simulink model "rsgTask"  (R2012b)
settings: Solver=FixedStepDiscrete  StartTime=0.0  StopTime=10.0  FixedStep=0.001  RelTol=1e-3
undefined symbols (not defined in the file): acquireMethods, autoplayMovementDuration, autoplayReactionTime, autoplayRotationDuration, autoplayRotationStart, centerOffset, clickPercentage, clickRefractoryPeriod, clickTargetColor, clickTargetHoverColor, clickTargs, coherences, contextIDs, contextTime, contextTimeVec, crossSize, cuedText, cuedTextLength, cumulativeDwell, cursorColorClick, cursorColorClosed, cursorColorOpen, cursorColors, cursorDiameter, cursorNeuralColor, cursorNonneuralColor, delayOrder, delayPeriodGainScale, delayTime, discreteOLMode, displayObject, doHeadSpeedFail, drawNumbersOnTargets, dwellRefractoryPeriod, errorAssistAxis, errorAssistR, errorAssistTheta, expRandBinSize, expRandMax, expRandMin, expRandMu, eyeMode, failOnLiftoff, failurePenalty, falseClickFails, fingerPositionTolerance, fixedSeqMode, freePlayMode, gain, gloveBias, gloveLPDenominator, gloveLPNumerator, gloveNonlinearCorrection, gloveXCorrection, gloveYCorrection, gracePeriod, gridEdges, gridSize, gridTilesEachDim, headSpeedCap ... (+133)
settings Model: Creator=gilja  LastModifiedBy=NPTL
settings SolverCC: EnableConcurrentExecution=on  ConcurrentTasks=on
settings DataIOCC: SaveOutput=off  SignalLogging=off  SaveTime=off
settings OptimizationCC: InlineParams=on  InlineInvariantSignals=on  EnhancedBackFolding=on  EfficientFloat2IntCast=on  SimCompilerOptimization=On
settings DebuggingCC: UnderspecifiedInitializationDetection=Simplified
settings HardwareCC: ProdIntDivRoundTo=Zero  ProdEndianess=LittleEndian  ProdHWDeviceType=Generic->32-bit x86 compatible
settings RTWCC: SystemTargetFile=xpctarget.tlc  TemplateMakefile=xpc_default_tmf  Description=xPC Target  ProcessScript=xpctarget_make_rtw_hook  RTWCompilerOptimization=On
settings CodeAppCC: MaxIdLength=62
settings xpcTargetCC: TargetFcnLib=ansi_tfl_table_tmw.mat  CodeReplacementLibrary=XPC_BLAS  ParMdlRefBuildCompliant=on  ConcurrentExecutionCompliant=on  CombineSignalStateStructs=off  GRTInterface=on  xPCTaskExecutionProfile=on  xPCRL32EventNumber=5000  xPCisDownloadable=off  xPCLoadParamSetFile=off  xPCConcurrentTasks=off  xPCEnableSFAnimation=off

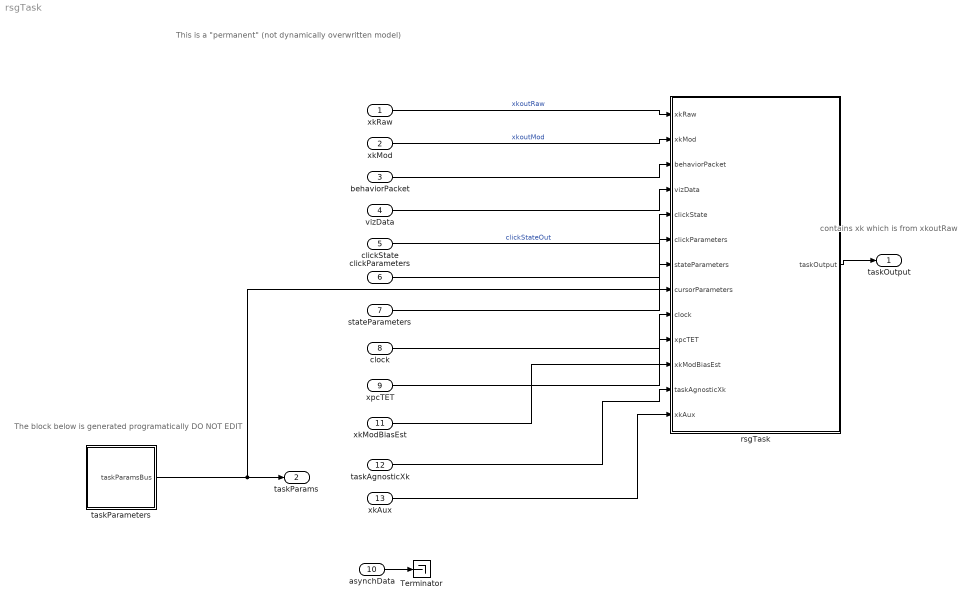
== system rsgTask ==
  note: contains xk which is
      | from xkoutRaw
  note: This is a "permanent" (not dynamically overwritten model)
  note: The block below is generated programatically
      | DO NOT EDIT
  xkRaw : Inport  OutDataTypeStr=double  PortDimensions=[double(xkConstants.NUM_STATE_DIMENSIONS),1]  SampleTime=[0.001,0]
  xkMod : Inport  Port=2  OutDataTypeStr=double  PortDimensions=[double(xkConstants.NUM_STATE_DIMENSIONS),1]  SampleTime=[0.001,0]
  behaviorPacket : Inport  Port=3  OutDataTypeStr=Bus: behaviorPacketBus  SampleTime=[0.001,0]
  vizData : Inport  Port=4  OutDataTypeStr=Bus: peripheralData  SampleTime=[0.001,0]
  clickState : Inport  Port=5  OutDataTypeStr=uint16  PortDimensions=1  SampleTime=[0.001,0]
  clickParameters : Inport  Port=6  OutDataTypeStr=Bus: clickParametersBus  SampleTime=[0.001,0]
  stateParameters : Inport  Port=7  OutDataTypeStr=Bus: stateParams  SampleTime=[0.001,0]
  clock : Inport  Port=8  OutDataTypeStr=uint32  PortDimensions=1  SampleTime=[0.001,0]
  xpcTET : Inport  Port=9  OutDataTypeStr=double  PortDimensions=1  SampleTime=[0.001,0]
  asynchData : Inport  Port=10  OutDataTypeStr=Bus: peripheralData  SampleTime=[0.001,0]
  xkModBiasEst : Inport  Port=11  OutDataTypeStr=double  PortDimensions=[double(xkConstants.NUM_STATE_DIMENSIONS),1]  SampleTime=[0.001,0]
  taskAgnosticXk : Inport  Port=12  OutDataTypeStr=double  PortDimensions=[double(xkConstants.NUM_STATE_DIMENSIONS),1]  SampleTime=[0.001,0]
  xkAux : Inport  Port=13  OutDataTypeStr=double  PortDimensions=[double(xkConstants.NUM_STATE_DIMENSIONS),1]  SampleTime=[0.001,0]
  Terminator : Terminator
  rsgTask : MATLAB Function  TreatAsAtomicUnit=on
  taskParameters : Subsystem
  taskOutput : Outport  OutDataTypeStr=Bus: taskOutput  PortDimensions=1  SampleTime=[0.001,0]  BusOutputAsStruct=on
  taskParams : Outport  Port=2  OutDataTypeStr=Bus: taskParamsBus  SampleTime=[0.001,0]
  wires:
  xkRaw/1 -> rsgTask/1(xkRaw)  "xkoutRaw"
  behaviorPacket/1 -> rsgTask/3(behaviorPacket)
  vizData/1 -> rsgTask/4(vizData)
  clickState/1 -> rsgTask/5(clickState)  "clickStateOut"
  clickParameters/1 -> rsgTask/6(clickParameters)
  clock/1 -> rsgTask/9(clock)
  xpcTET/1 -> rsgTask/10(xpcTET)
  stateParameters/1 -> rsgTask/7(stateParameters)
  taskParameters/1(taskParamsBus) -> taskParams/1, rsgTask/8(cursorParameters)
  rsgTask/1(taskOutput) -> taskOutput/1
  asynchData/1 -> Terminator/1
  xkMod/1 -> rsgTask/2(xkMod)  "xkoutMod"
  xkModBiasEst/1 -> rsgTask/11(xkModBiasEst)
  taskAgnosticXk/1 -> rsgTask/12(taskAgnosticXk)
  xkAux/1 -> rsgTask/13(xkAux)

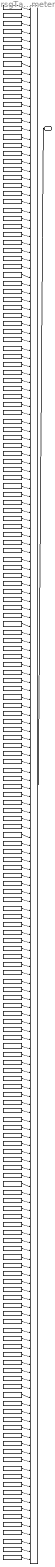
== system rsgTask/taskParameters ==
  BusOutput : BusCreator  Inputs=targetDiameter,maxTaskTime,holdTime,trialTimeout,numTrials,randomSeed,expRandMu,expRandMin,expRandMax,expRandBinSize,taskType,targetInds,numTargets,gain,failurePenalty,cursorDiameter,inputType,gloveBias,useRandomDelay,mouseOffset,workspaceX,workspaceY,workspaceZ,workspaceR,workspaceR2,showScores,trialsPerScore,cursorColorClick,recenterOnFail,recenterOnSuccess,recenterDelay,initialInput,clickPercentage,lockFingerPosition,fingerPositionTolerance,failOnLiftoff,errorAssistR,errorAssistTheta,errorAssistAxis,useGloveLPF,gloveLPNumerator,gloveLPDenominator,gloveNonlinearCorrection,gloveYCorrection,gloveXCorrection,useMouseLPF,soundOnFail,soundOnGo,soundOnSuccess,soundOnOverTarget,mouseLPNumerator,mouseLPDenominator,stopOffTarget,stopOnClick,outputType,xk2HorizontalPos,xk2HorizontalVel,xk2VerticalPos,xk2VerticalVel,xk2DepthPos,xk2DepthVel,xk2RotatePos,xk2RotateVel,xk2Rotate2Pos,xk2Rotate2Vel,gridEdges,gridTilesEachDim,selectionRefractoryMS,autoplayReactionTime,autoplayMovementDuration,powerGain,powerGainUnityCrossing,targetRotDiameter,autoplayRotationStart,autoplayRotationDuration,randomTaskTargetDiameters,randomTaskTargetRotDiameters,randomTaskBoundaries,numDisplayDims,cursorColorOpen,cursorColorClosed,showXYZaura,displayObject,preTrialLength,targetDiameters,numTargetDiameters,minTargetDistance,targetDelay,targetSpaceX,targetSpaceY,clickTargetColor,clickTargetHoverColor,falseClickFails,splitDimensions,vmrTheta,doHeadSpeedFail,headSpeedCap,eyeMode,speedTaskMode,delayPeriodGainScale,wiaMode,showWiaText,freePlayMode,drawNumbersOnTargets,xkRawSpeedCap,discreteOLMode,movementDuration,holdDuration,restDuration,returnDuration,repsPerBlock,whichMovements,movementOrder,delayOrder,textOverlayID,clickRefractoryPeriod,xpcVelocityOutputPeriodMS,outputVelocityScaling,screenUpdateRate,targetDevice,playSpokenCues,numTargetsInSeq,targetSeq,seqReadyTime,seqRehearseTime,rotateSeqCues,numRepsPerSeq,rehearsalOrder,rehearsalTimes,pathMode,memorizeMode,fixedSeqMode,sequenceMatrix,keyboard,resetDisplay,cursorNeuralColor,cursorNonneuralColor,centerOffset,scoreTime,cuedTextLength,cuedText,keyboardDims,recenterFullscreen,soundOnError,acquireMethods,cumulativeDwell,showBackspace,showStartStop,showTargetText,showTypedText,showCueOnTarget,showCueOffTarget,recenterOffset,dwellRefractoryPeriod,keyPressedTime,initialLockout,initialState,symbolMoveTimeOne,symbolRehearseTime,symbolGetReadyTime,symbolMoveTimeTwo,symbolVMRMode,symbolVMRRot,pc1MouseInControlMode,gracePeriod,maxFixDur,maxTargDur,maxStimDur,moveThresh,intertrialTime,cursorColors,gridSize,crossSize,makeGrid,tau,taskOrder,stimDur,coherences,contextIDs,stimConds,contextTime,stimTime,delayTime,contextTimeVec,nextClickTarg,clickTargs,rsgTargetSeq,rsgTargetLoc,rsgCueDisplayTime,rsgProductionTimes,rsgPreReadyTimes,rsgFixationRadius  OutDataTypeStr=Bus: taskParamsBus
  acquireMethods : Constant  Value=acquireMethods
  autoplayMovementDuration : Constant  Value=autoplayMovementDuration
  autoplayReactionTime : Constant  Value=autoplayReactionTime
  autoplayRotationDuration : Constant  Value=autoplayRotationDuration
  autoplayRotationStart : Constant  Value=autoplayRotationStart
  centerOffset : Constant  Value=centerOffset
  clickPercentage : Constant  Value=clickPercentage
  clickRefractoryPeriod : Constant  Value=clickRefractoryPeriod
  clickTargetColor : Constant  Value=clickTargetColor
  clickTargetHoverColor : Constant  Value=clickTargetHoverColor
  clickTargs : Constant  Value=clickTargs
  coherences : Constant  Value=coherences
  contextIDs : Constant  Value=contextIDs
  contextTime : Constant  Value=contextTime
  contextTimeVec : Constant  Value=contextTimeVec
  crossSize : Constant  Value=crossSize
  cuedText : Constant  Value=cuedText
  cuedTextLength : Constant  Value=cuedTextLength
  cumulativeDwell : Constant  Value=cumulativeDwell
  cursorColorClick : Constant  Value=cursorColorClick
  cursorColorClosed : Constant  Value=cursorColorClosed
  cursorColorOpen : Constant  Value=cursorColorOpen
  cursorColors : Constant  Value=cursorColors
  cursorDiameter : Constant  Value=cursorDiameter
  cursorNeuralColor : Constant  Value=cursorNeuralColor
  cursorNonneuralColor : Constant  Value=cursorNonneuralColor
  delayOrder : Constant  Value=delayOrder
  delayPeriodGainScale : Constant  Value=delayPeriodGainScale
  delayTime : Constant  Value=delayTime
  discreteOLMode : Constant  Value=discreteOLMode
  displayObject : Constant  Value=displayObject
  doHeadSpeedFail : Constant  Value=doHeadSpeedFail
  drawNumbersOnTargets : Constant  Value=drawNumbersOnTargets
  dwellRefractoryPeriod : Constant  Value=dwellRefractoryPeriod
  errorAssistAxis : Constant  Value=errorAssistAxis
  errorAssistR : Constant  Value=errorAssistR
  errorAssistTheta : Constant  Value=errorAssistTheta
  expRandBinSize : Constant  Value=expRandBinSize
  expRandMax : Constant  Value=expRandMax
  expRandMin : Constant  Value=expRandMin
  expRandMu : Constant  Value=expRandMu
  eyeMode : Constant  Value=eyeMode
  failOnLiftoff : Constant  Value=failOnLiftoff
  failurePenalty : Constant  Value=failurePenalty
  falseClickFails : Constant  Value=falseClickFails
  fingerPositionTolerance : Constant  Value=fingerPositionTolerance
  fixedSeqMode : Constant  Value=fixedSeqMode
  freePlayMode : Constant  Value=freePlayMode
  gain : Constant  Value=gain
  gloveBias : Constant  Value=gloveBias
  gloveLPDenominator : Constant  Value=gloveLPDenominator
  gloveLPNumerator : Constant  Value=gloveLPNumerator
  gloveNonlinearCorrection : Constant  Value=gloveNonlinearCorrection
  gloveXCorrection : Constant  Value=gloveXCorrection
  gloveYCorrection : Constant  Value=gloveYCorrection
  gracePeriod : Constant  Value=gracePeriod
  gridEdges : Constant  Value=gridEdges
  gridSize : Constant  Value=gridSize
  gridTilesEachDim : Constant  Value=gridTilesEachDim
  headSpeedCap : Constant  Value=headSpeedCap
  holdDuration : Constant  Value=holdDuration
  holdTime : Constant  Value=holdTime
  initialInput : Constant  Value=initialInput
  initialLockout : Constant  Value=initialLockout
  initialState : Constant  Value=initialState
  inputType : Constant  Value=inputType
  intertrialTime : Constant  Value=intertrialTime
  keyPressedTime : Constant  Value=keyPressedTime
  keyboard : Constant  Value=keyboard
  keyboardDims : Constant  Value=keyboardDims
  lockFingerPosition : Constant  Value=lockFingerPosition
  makeGrid : Constant  Value=makeGrid
  maxFixDur : Constant  Value=maxFixDur
  maxStimDur : Constant  Value=maxStimDur
  maxTargDur : Constant  Value=maxTargDur
  maxTaskTime : Constant  Value=maxTaskTime
  memorizeMode : Constant  Value=memorizeMode
  minTargetDistance : Constant  Value=minTargetDistance
  mouseLPDenominator : Constant  Value=mouseLPDenominator
  mouseLPNumerator : Constant  Value=mouseLPNumerator
  mouseOffset : Constant  Value=mouseOffset
  moveThresh : Constant  Value=moveThresh
  movementDuration : Constant  Value=movementDuration
  movementOrder : Constant  Value=movementOrder
  nextClickTarg : Constant  Value=nextClickTarg
  numDisplayDims : Constant  Value=numDisplayDims
  numRepsPerSeq : Constant  Value=numRepsPerSeq
  numTargetDiameters : Constant  Value=numTargetDiameters
  numTargets : Constant  Value=numTargets
  numTargetsInSeq : Constant  Value=numTargetsInSeq
  numTrials : Constant  Value=numTrials
  outputType : Constant  Value=outputType
  outputVelocityScaling : Constant  Value=outputVelocityScaling
  pathMode : Constant  Value=pathMode
  pc1MouseInControlMode : Constant  Value=pc1MouseInControlMode
  playSpokenCues : Constant  Value=playSpokenCues
  powerGain : Constant  Value=powerGain
  powerGainUnityCrossing : Constant  Value=powerGainUnityCrossing
  preTrialLength : Constant  Value=preTrialLength
  randomSeed : Constant  Value=randomSeed
  randomTaskBoundaries : Constant  Value=randomTaskBoundaries
  randomTaskTargetDiameters : Constant  Value=randomTaskTargetDiameters
  randomTaskTargetRotDiameters : Constant  Value=randomTaskTargetRotDiameters
  recenterDelay : Constant  Value=recenterDelay
  recenterFullscreen : Constant  Value=recenterFullscreen
  recenterOffset : Constant  Value=recenterOffset
  recenterOnFail : Constant  Value=recenterOnFail
  recenterOnSuccess : Constant  Value=recenterOnSuccess
  rehearsalOrder : Constant  Value=rehearsalOrder
  rehearsalTimes : Constant  Value=rehearsalTimes
  repsPerBlock : Constant  Value=repsPerBlock
  resetDisplay : Constant  Value=resetDisplay
  restDuration : Constant  Value=restDuration
  returnDuration : Constant  Value=returnDuration
  rotateSeqCues : Constant  Value=rotateSeqCues
  rsgCueDisplayTime : Constant  Value=rsgCueDisplayTime
  rsgFixationRadius : Constant  Value=rsgFixationRadius
  rsgPreReadyTimes : Constant  Value=rsgPreReadyTimes
  rsgProductionTimes : Constant  Value=rsgProductionTimes
  rsgTargetLoc : Constant  Value=rsgTargetLoc
  rsgTargetSeq : Constant  Value=rsgTargetSeq
  scoreTime : Constant  Value=scoreTime
  screenUpdateRate : Constant  Value=screenUpdateRate
  selectionRefractoryMS : Constant  Value=selectionRefractoryMS
  seqReadyTime : Constant  Value=seqReadyTime
  seqRehearseTime : Constant  Value=seqRehearseTime
  sequenceMatrix : Constant  Value=sequenceMatrix
  showBackspace : Constant  Value=showBackspace
  showCueOffTarget : Constant  Value=showCueOffTarget
  showCueOnTarget : Constant  Value=showCueOnTarget
  showScores : Constant  Value=showScores
  showStartStop : Constant  Value=showStartStop
  showTargetText : Constant  Value=showTargetText
  showTypedText : Constant  Value=showTypedText
  showWiaText : Constant  Value=showWiaText
  showXYZaura : Constant  Value=showXYZaura
  soundOnError : Constant  Value=soundOnError
  soundOnFail : Constant  Value=soundOnFail
  soundOnGo : Constant  Value=soundOnGo
  soundOnOverTarget : Constant  Value=soundOnOverTarget
  soundOnSuccess : Constant  Value=soundOnSuccess
  speedTaskMode : Constant  Value=speedTaskMode
  splitDimensions : Constant  Value=splitDimensions
  stimConds : Constant  Value=stimConds
  stimDur : Constant  Value=stimDur
  stimTime : Constant  Value=stimTime
  stopOffTarget : Constant  Value=stopOffTarget
  stopOnClick : Constant  Value=stopOnClick
  symbolGetReadyTime : Constant  Value=symbolGetReadyTime
  symbolMoveTimeOne : Constant  Value=symbolMoveTimeOne
  symbolMoveTimeTwo : Constant  Value=symbolMoveTimeTwo
  symbolRehearseTime : Constant  Value=symbolRehearseTime
  symbolVMRMode : Constant  Value=symbolVMRMode
  symbolVMRRot : Constant  Value=symbolVMRRot
  targetDelay : Constant  Value=targetDelay
  targetDevice : Constant  Value=targetDevice
  targetDiameter : Constant  Value=targetDiameter
  targetDiameters : Constant  Value=targetDiameters
  targetInds : Constant  Value=targetInds
  targetRotDiameter : Constant  Value=targetRotDiameter
  targetSeq : Constant  Value=targetSeq
  targetSpaceX : Constant  Value=targetSpaceX
  targetSpaceY : Constant  Value=targetSpaceY
  taskOrder : Constant  Value=taskOrder
  taskType : Constant  Value=taskType
  tau : Constant  Value=tau
  textOverlayID : Constant  Value=textOverlayID
  trialTimeout : Constant  Value=trialTimeout
  trialsPerScore : Constant  Value=trialsPerScore
  useGloveLPF : Constant  Value=useGloveLPF
  useMouseLPF : Constant  Value=useMouseLPF
  useRandomDelay : Constant  Value=useRandomDelay
  vmrTheta : Constant  Value=vmrTheta
  whichMovements : Constant  Value=whichMovements
  wiaMode : Constant  Value=wiaMode
  workspaceR : Constant  Value=workspaceR
  workspaceR2 : Constant  Value=workspaceR2
  workspaceX : Constant  Value=workspaceX
  workspaceY : Constant  Value=workspaceY
  workspaceZ : Constant  Value=workspaceZ
  xk2DepthPos : Constant  Value=xk2DepthPos
  xk2DepthVel : Constant  Value=xk2DepthVel
  xk2HorizontalPos : Constant  Value=xk2HorizontalPos
  xk2HorizontalVel : Constant  Value=xk2HorizontalVel
  xk2Rotate2Pos : Constant  Value=xk2Rotate2Pos
  xk2Rotate2Vel : Constant  Value=xk2Rotate2Vel
  xk2RotatePos : Constant  Value=xk2RotatePos
  xk2RotateVel : Constant  Value=xk2RotateVel
  xk2VerticalPos : Constant  Value=xk2VerticalPos
  xk2VerticalVel : Constant  Value=xk2VerticalVel
  xkRawSpeedCap : Constant  Value=xkRawSpeedCap
  xpcVelocityOutputPeriodMS : Constant  Value=xpcVelocityOutputPeriodMS
  taskParamsBus : Outport
  wires:
  targetDiameter/1 -> BusOutput/1  "targetDiameter"
  maxTaskTime/1 -> BusOutput/2  "maxTaskTime"
  holdTime/1 -> BusOutput/3  "holdTime"
  trialTimeout/1 -> BusOutput/4  "trialTimeout"
  numTrials/1 -> BusOutput/5  "numTrials"
  randomSeed/1 -> BusOutput/6  "randomSeed"
  expRandMu/1 -> BusOutput/7  "expRandMu"
  expRandMin/1 -> BusOutput/8  "expRandMin"
  expRandMax/1 -> BusOutput/9  "expRandMax"
  expRandBinSize/1 -> BusOutput/10  "expRandBinSize"
  taskType/1 -> BusOutput/11  "taskType"
  targetInds/1 -> BusOutput/12  "targetInds"
  numTargets/1 -> BusOutput/13  "numTargets"
  gain/1 -> BusOutput/14  "gain"
  failurePenalty/1 -> BusOutput/15  "failurePenalty"
  cursorDiameter/1 -> BusOutput/16  "cursorDiameter"
  inputType/1 -> BusOutput/17  "inputType"
  gloveBias/1 -> BusOutput/18  "gloveBias"
  useRandomDelay/1 -> BusOutput/19  "useRandomDelay"
  mouseOffset/1 -> BusOutput/20  "mouseOffset"
  workspaceX/1 -> BusOutput/21  "workspaceX"
  workspaceY/1 -> BusOutput/22  "workspaceY"
  workspaceZ/1 -> BusOutput/23  "workspaceZ"
  workspaceR/1 -> BusOutput/24  "workspaceR"
  workspaceR2/1 -> BusOutput/25  "workspaceR2"
  showScores/1 -> BusOutput/26  "showScores"
  trialsPerScore/1 -> BusOutput/27  "trialsPerScore"
  cursorColorClick/1 -> BusOutput/28  "cursorColorClick"
  recenterOnFail/1 -> BusOutput/29  "recenterOnFail"
  recenterOnSuccess/1 -> BusOutput/30  "recenterOnSuccess"
  recenterDelay/1 -> BusOutput/31  "recenterDelay"
  initialInput/1 -> BusOutput/32  "initialInput"
  clickPercentage/1 -> BusOutput/33  "clickPercentage"
  lockFingerPosition/1 -> BusOutput/34  "lockFingerPosition"
  fingerPositionTolerance/1 -> BusOutput/35  "fingerPositionTolerance"
  failOnLiftoff/1 -> BusOutput/36  "failOnLiftoff"
  errorAssistR/1 -> BusOutput/37  "errorAssistR"
  errorAssistTheta/1 -> BusOutput/38  "errorAssistTheta"
  errorAssistAxis/1 -> BusOutput/39  "errorAssistAxis"
  useGloveLPF/1 -> BusOutput/40  "useGloveLPF"
  gloveLPNumerator/1 -> BusOutput/41  "gloveLPNumerator"
  gloveLPDenominator/1 -> BusOutput/42  "gloveLPDenominator"
  gloveNonlinearCorrection/1 -> BusOutput/43  "gloveNonlinearCorrection"
  gloveYCorrection/1 -> BusOutput/44  "gloveYCorrection"
  gloveXCorrection/1 -> BusOutput/45  "gloveXCorrection"
  useMouseLPF/1 -> BusOutput/46  "useMouseLPF"
  soundOnFail/1 -> BusOutput/47  "soundOnFail"
  soundOnGo/1 -> BusOutput/48  "soundOnGo"
  soundOnSuccess/1 -> BusOutput/49  "soundOnSuccess"
  soundOnOverTarget/1 -> BusOutput/50  "soundOnOverTarget"
  mouseLPNumerator/1 -> BusOutput/51  "mouseLPNumerator"
  mouseLPDenominator/1 -> BusOutput/52  "mouseLPDenominator"
  stopOffTarget/1 -> BusOutput/53  "stopOffTarget"
  stopOnClick/1 -> BusOutput/54  "stopOnClick"
  outputType/1 -> BusOutput/55  "outputType"
  xk2HorizontalPos/1 -> BusOutput/56  "xk2HorizontalPos"
  xk2HorizontalVel/1 -> BusOutput/57  "xk2HorizontalVel"
  xk2VerticalPos/1 -> BusOutput/58  "xk2VerticalPos"
  xk2VerticalVel/1 -> BusOutput/59  "xk2VerticalVel"
  xk2DepthPos/1 -> BusOutput/60  "xk2DepthPos"
  xk2DepthVel/1 -> BusOutput/61  "xk2DepthVel"
  xk2RotatePos/1 -> BusOutput/62  "xk2RotatePos"
  xk2RotateVel/1 -> BusOutput/63  "xk2RotateVel"
  xk2Rotate2Pos/1 -> BusOutput/64  "xk2Rotate2Pos"
  xk2Rotate2Vel/1 -> BusOutput/65  "xk2Rotate2Vel"
  gridEdges/1 -> BusOutput/66  "gridEdges"
  gridTilesEachDim/1 -> BusOutput/67  "gridTilesEachDim"
  selectionRefractoryMS/1 -> BusOutput/68  "selectionRefractoryMS"
  autoplayReactionTime/1 -> BusOutput/69  "autoplayReactionTime"
  autoplayMovementDuration/1 -> BusOutput/70  "autoplayMovementDuration"
  powerGain/1 -> BusOutput/71  "powerGain"
  powerGainUnityCrossing/1 -> BusOutput/72  "powerGainUnityCrossing"
  targetRotDiameter/1 -> BusOutput/73  "targetRotDiameter"
  autoplayRotationStart/1 -> BusOutput/74  "autoplayRotationStart"
  autoplayRotationDuration/1 -> BusOutput/75  "autoplayRotationDuration"
  randomTaskTargetDiameters/1 -> BusOutput/76  "randomTaskTargetDiameters"
  randomTaskTargetRotDiameters/1 -> BusOutput/77  "randomTaskTargetRotDiameters"
  randomTaskBoundaries/1 -> BusOutput/78  "randomTaskBoundaries"
  numDisplayDims/1 -> BusOutput/79  "numDisplayDims"
  cursorColorOpen/1 -> BusOutput/80  "cursorColorOpen"
  cursorColorClosed/1 -> BusOutput/81  "cursorColorClosed"
  showXYZaura/1 -> BusOutput/82  "showXYZaura"
  displayObject/1 -> BusOutput/83  "displayObject"
  preTrialLength/1 -> BusOutput/84  "preTrialLength"
  targetDiameters/1 -> BusOutput/85  "targetDiameters"
  numTargetDiameters/1 -> BusOutput/86  "numTargetDiameters"
  minTargetDistance/1 -> BusOutput/87  "minTargetDistance"
  targetDelay/1 -> BusOutput/88  "targetDelay"
  targetSpaceX/1 -> BusOutput/89  "targetSpaceX"
  targetSpaceY/1 -> BusOutput/90  "targetSpaceY"
  clickTargetColor/1 -> BusOutput/91  "clickTargetColor"
  clickTargetHoverColor/1 -> BusOutput/92  "clickTargetHoverColor"
  falseClickFails/1 -> BusOutput/93  "falseClickFails"
  splitDimensions/1 -> BusOutput/94  "splitDimensions"
  vmrTheta/1 -> BusOutput/95  "vmrTheta"
  doHeadSpeedFail/1 -> BusOutput/96  "doHeadSpeedFail"
  headSpeedCap/1 -> BusOutput/97  "headSpeedCap"
  eyeMode/1 -> BusOutput/98  "eyeMode"
  speedTaskMode/1 -> BusOutput/99  "speedTaskMode"
  delayPeriodGainScale/1 -> BusOutput/100  "delayPeriodGainScale"
  wiaMode/1 -> BusOutput/101  "wiaMode"
  showWiaText/1 -> BusOutput/102  "showWiaText"
  freePlayMode/1 -> BusOutput/103  "freePlayMode"
  drawNumbersOnTargets/1 -> BusOutput/104  "drawNumbersOnTargets"
  xkRawSpeedCap/1 -> BusOutput/105  "xkRawSpeedCap"
  discreteOLMode/1 -> BusOutput/106  "discreteOLMode"
  movementDuration/1 -> BusOutput/107  "movementDuration"
  holdDuration/1 -> BusOutput/108  "holdDuration"
  restDuration/1 -> BusOutput/109  "restDuration"
  returnDuration/1 -> BusOutput/110  "returnDuration"
  repsPerBlock/1 -> BusOutput/111  "repsPerBlock"
  whichMovements/1 -> BusOutput/112  "whichMovements"
  movementOrder/1 -> BusOutput/113  "movementOrder"
  delayOrder/1 -> BusOutput/114  "delayOrder"
  textOverlayID/1 -> BusOutput/115  "textOverlayID"
  clickRefractoryPeriod/1 -> BusOutput/116  "clickRefractoryPeriod"
  xpcVelocityOutputPeriodMS/1 -> BusOutput/117  "xpcVelocityOutputPeriodMS"
  outputVelocityScaling/1 -> BusOutput/118  "outputVelocityScaling"
  screenUpdateRate/1 -> BusOutput/119  "screenUpdateRate"
  targetDevice/1 -> BusOutput/120  "targetDevice"
  playSpokenCues/1 -> BusOutput/121  "playSpokenCues"
  numTargetsInSeq/1 -> BusOutput/122  "numTargetsInSeq"
  targetSeq/1 -> BusOutput/123  "targetSeq"
  seqReadyTime/1 -> BusOutput/124  "seqReadyTime"
  seqRehearseTime/1 -> BusOutput/125  "seqRehearseTime"
  rotateSeqCues/1 -> BusOutput/126  "rotateSeqCues"
  numRepsPerSeq/1 -> BusOutput/127  "numRepsPerSeq"
  rehearsalOrder/1 -> BusOutput/128  "rehearsalOrder"
  rehearsalTimes/1 -> BusOutput/129  "rehearsalTimes"
  pathMode/1 -> BusOutput/130  "pathMode"
  memorizeMode/1 -> BusOutput/131  "memorizeMode"
  fixedSeqMode/1 -> BusOutput/132  "fixedSeqMode"
  sequenceMatrix/1 -> BusOutput/133  "sequenceMatrix"
  keyboard/1 -> BusOutput/134  "keyboard"
  resetDisplay/1 -> BusOutput/135  "resetDisplay"
  cursorNeuralColor/1 -> BusOutput/136  "cursorNeuralColor"
  cursorNonneuralColor/1 -> BusOutput/137  "cursorNonneuralColor"
  centerOffset/1 -> BusOutput/138  "centerOffset"
  scoreTime/1 -> BusOutput/139  "scoreTime"
  cuedTextLength/1 -> BusOutput/140  "cuedTextLength"
  cuedText/1 -> BusOutput/141  "cuedText"
  keyboardDims/1 -> BusOutput/142  "keyboardDims"
  recenterFullscreen/1 -> BusOutput/143  "recenterFullscreen"
  soundOnError/1 -> BusOutput/144  "soundOnError"
  acquireMethods/1 -> BusOutput/145  "acquireMethods"
  cumulativeDwell/1 -> BusOutput/146  "cumulativeDwell"
  showBackspace/1 -> BusOutput/147  "showBackspace"
  showStartStop/1 -> BusOutput/148  "showStartStop"
  showTargetText/1 -> BusOutput/149  "showTargetText"
  showTypedText/1 -> BusOutput/150  "showTypedText"
  showCueOnTarget/1 -> BusOutput/151  "showCueOnTarget"
  showCueOffTarget/1 -> BusOutput/152  "showCueOffTarget"
  recenterOffset/1 -> BusOutput/153  "recenterOffset"
  dwellRefractoryPeriod/1 -> BusOutput/154  "dwellRefractoryPeriod"
  keyPressedTime/1 -> BusOutput/155  "keyPressedTime"
  initialLockout/1 -> BusOutput/156  "initialLockout"
  initialState/1 -> BusOutput/157  "initialState"
  symbolMoveTimeOne/1 -> BusOutput/158  "symbolMoveTimeOne"
  symbolRehearseTime/1 -> BusOutput/159  "symbolRehearseTime"
  symbolGetReadyTime/1 -> BusOutput/160  "symbolGetReadyTime"
  symbolMoveTimeTwo/1 -> BusOutput/161  "symbolMoveTimeTwo"
  symbolVMRMode/1 -> BusOutput/162  "symbolVMRMode"
  symbolVMRRot/1 -> BusOutput/163  "symbolVMRRot"
  pc1MouseInControlMode/1 -> BusOutput/164  "pc1MouseInControlMode"
  gracePeriod/1 -> BusOutput/165  "gracePeriod"
  maxFixDur/1 -> BusOutput/166  "maxFixDur"
  maxTargDur/1 -> BusOutput/167  "maxTargDur"
  maxStimDur/1 -> BusOutput/168  "maxStimDur"
  moveThresh/1 -> BusOutput/169  "moveThresh"
  intertrialTime/1 -> BusOutput/170  "intertrialTime"
  cursorColors/1 -> BusOutput/171  "cursorColors"
  gridSize/1 -> BusOutput/172  "gridSize"
  crossSize/1 -> BusOutput/173  "crossSize"
  makeGrid/1 -> BusOutput/174  "makeGrid"
  tau/1 -> BusOutput/175  "tau"
  taskOrder/1 -> BusOutput/176  "taskOrder"
  stimDur/1 -> BusOutput/177  "stimDur"
  coherences/1 -> BusOutput/178  "coherences"
  contextIDs/1 -> BusOutput/179  "contextIDs"
  stimConds/1 -> BusOutput/180  "stimConds"
  contextTime/1 -> BusOutput/181  "contextTime"
  stimTime/1 -> BusOutput/182  "stimTime"
  delayTime/1 -> BusOutput/183  "delayTime"
  contextTimeVec/1 -> BusOutput/184  "contextTimeVec"
  nextClickTarg/1 -> BusOutput/185  "nextClickTarg"
  clickTargs/1 -> BusOutput/186  "clickTargs"
  rsgTargetSeq/1 -> BusOutput/187  "rsgTargetSeq"
  rsgTargetLoc/1 -> BusOutput/188  "rsgTargetLoc"
  rsgCueDisplayTime/1 -> BusOutput/189  "rsgCueDisplayTime"
  rsgProductionTimes/1 -> BusOutput/190  "rsgProductionTimes"
  rsgPreReadyTimes/1 -> BusOutput/191  "rsgPreReadyTimes"
  rsgFixationRadius/1 -> BusOutput/192  "rsgFixationRadius"
  BusOutput/1 -> taskParamsBus/1

== matlab function rsgTask/rsgTask ==
  data: xkRaw input double size=[double(xkConstants.NUM_STATE_DIMENSIONS) 1]; xkMod input; behaviorPacket input Bus: behaviorPacketBus size=1; vizData input Bus: peripheralData; clickState input; clickParameters input; taskOutput output Bus: taskOutput; stateParameters input Bus: stateParams size=1; cursorParameters input Bus: taskParamsBus; clock input; xpcTET input; xkModBiasEst input; taskAgnosticXk input; xkAux input
function taskOutput  = rsgTask(xkRaw, xkMod, behaviorPacket, vizData, clickState, clickParameters, ...
    stateParameters, cursorParameters, clock, xpcTET, xkModBiasEst, taskAgnosticXk, xkAux)

%#codegen
behaviorRequestClock = behaviorPacket.xpcRequestClock;
peripheralTimestamp = behaviorPacket.peripheralTimestamp(1:16);

%% CONSTANTS
TASK_NAME = 'rsg';
VERSION_ID = single(1.0);

%% INITIALIZE CURSOR TASK OUTPUT
fileLoggerData.data = uint8(zeros(1,1400));
fileLoggerData.dataLen = uint16(0);
fileLoggerData.fileName = uint8(zeros(1,20));
fileLoggerData.send = false;

fileLoggerFormat.format = uint8(zeros(1,1400));
fileLoggerFormat.formatLen = uint16(0);
fileLoggerFormat.fileName = uint8(zeros(1,20));

fileLoggerFormatAndData.format = fileLoggerFormat;
fileLoggerFormatAndData.data = fileLoggerData;

taskOutput.flushFiles = false;
taskOutput.sendFormat = false;
taskOutput.taskDetails = fileLoggerFormat;
taskOutput.discrete = fileLoggerFormatAndData;
taskOutput.continuous = fileLoggerFormatAndData;
taskOutput.screen = fileLoggerFormatAndData;
taskOutput.sound = fileLoggerFormatAndData;
taskOutput.asynch = fileLoggerFormatAndData;
taskOutput.ttl = double(0);
taskOutput.xk = xkRaw;
taskOutput.inputType = cursorParameters.inputType;
taskOutput.currentTarget = single(zeros([double(xkConstants.NUM_TARGET_DIMENSIONS) 1]));
taskOutput.state = uint16(SequenceStates.STATE_MOVE);
taskOutput.paused = false;
taskOutput.allowStop = true;
taskOutput.resetHMM = true;

%% TASK DETAILS PACKET
taskOutput.taskDetails = packFileLoggerTaskDetails(TASK_NAME, VERSION_ID, ...
    'STATE_INIT', uint8(rsgStates.STATE_INIT), ...
    'STATE_FIXATE', uint8(rsgStates.STATE_FIXATE),...
    'STATE_PRE_READY', uint8(rsgStates.STATE_PRE_READY),...
    'STATE_POST_READY', uint8(rsgStates.STATE_POST_READY), ...
    'STATE_POST_SET', uint8(rsgStates.STATE_POST_SET),...
    'STATE_ACQUIRE', uint8(rsgStates.STATE_ACQUIRE),...
    'INPUT_TYPE_DECODE_V', uint8(cursorConstants.INPUT_TYPE_DECODE_V),...
    'INPUT_TYPE_HEAD_MOUSE', uint8(cursorConstants.INPUT_TYPE_HEAD_MOUSE) ...
);

%% DEFINE PERSISTENTS
persistent holdTimer 
persistent stateTimer;
persistent trialIdx;
persistent avgErr;
persistent totalErr;
persistent percentErr;
persistent state;

persistent lastSoundTime;
persistent lastSoundState;
persistent vizPacket;
persistent pastPause;

persistent prevHeadPos;
persistent filteredHeadSpeed;

persistent err;
persistent producedTime;
persistent currentTargIdx;

%% INITIALIZE PERSISTENTS
if(isempty(holdTimer))
    holdTimer = uint16(0);
    stateTimer = uint32(0);
    trialIdx = uint32(1);
    avgErr = single(0);
    totalErr = single(0);
    currentTargIdx = uint32(1);

    state = uint8(rsgStates.STATE_INIT);
    prevHeadPos = single(zeros(2,1));
    filteredHeadSpeed = single(0);

    lastSoundTime = clock;
    lastSoundState = uint8(SequenceStates.SOUND_STATE_IDLE);

    vizPacket = initVizPacket();
    pastPause = false;
    
    err = int32(-5000);
    producedTime = int32(-5000);
end
inputType = cursorParameters.inputType;

%% some initialization
outputType = cursorParameters.outputType; % determines what graphics engine will render this task.

writeDiscreteData = false;
writeContinuousData = true;

if(vizData.receive && (vizData.dataLen > 0 ))
    vizPacket = parseVizPacket(vizData.data);
end

effectorPos = zeros(1,2);
effectorPos(1) = behaviorPacket.windowsMousePosition(1)*1080;
effectorPos(2) = -behaviorPacket.windowsMousePosition(2)*1080;

INIT_TIME = uint32(2000);
pauseToggled = (pastPause==true) && (stateParameters.pause==false);
pauseTriggered = stateParameters.pause;
pastPause = stateParameters.pause;

if(clock < INIT_TIME)
    state = uint8(rsgStates.STATE_INIT);
    pauseTriggered = true;
elseif (state == uint8(rsgStates.STATE_INIT)) && pauseToggled
    state = uint8(rsgStates.STATE_FIXATE);
    stateTimer = uint32(1);
    trialIdx = uint32(0);
end

%%
%continuously affect state of RNG so we get somewhat random numbers from
%run to run
junkVal = rand(1,1);

%%
%estimate movement speed
headSpeedAlpha = single(0.96);
headSpeed = 1000*sqrt(sum((behaviorPacket.windowsMousePosition - prevHeadPos).^2));
filteredHeadSpeed = headSpeedAlpha*filteredHeadSpeed + (1-headSpeedAlpha)*headSpeed;
prevHeadPos = behaviorPacket.windowsMousePosition;

%%
%trial initialization
if (state == uint8(rsgStates.STATE_FIXATE)) && stateTimer==1
    trialIdx = trialIdx + 1;
    currentTargIdx = uint32(cursorParameters.rsgTargetSeq(trialIdx));
    
    err = int32(-5000);
    producedTime = int32(-5000);
end

%%
%manage target acquisition logic for whatever "target" (fixation center or actual target) may be active
targPos = single(cursorParameters.rsgTargetLoc(1:2,currentTargIdx)');
acquiredTarget = false;
targOverlap = false;

if (state == uint8(rsgStates.STATE_FIXATE)) || (state == uint8(rsgStates.STATE_ACQUIRE))
    holdLogicTargPos = single(zeros(1,2));
    effectiveRadius = single(0);
    if (state == uint8(rsgStates.STATE_FIXATE))
        holdLogicTargPos = single(zeros(1,2));
        effectiveRadius = cursorParameters.rsgFixationRadius;
    elseif (state == uint8(rsgStates.STATE_ACQUIRE))
        holdLogicTargPos = targPos;
        effectiveRadius = (cursorParameters.targetDiameter + cursorParameters.cursorDiameter)/2;
    end

    targDist = single(sqrt(sum((effectorPos - holdLogicTargPos).^2)));
    targOverlap = targDist < effectiveRadius;

    if targOverlap
        holdTimer = holdTimer + 1;
    else
        holdTimer = uint16(0);
    end
    if holdTimer > cursorParameters.holdTime
        %target acquired
        holdTimer = uint16(0);
        acquiredTarget = true;
    else
        acquiredTarget = false;
    end
end

%%
%trigger state transitions based on target acquisition
if (state == uint8(rsgStates.STATE_FIXATE)) && acquiredTarget
    state = uint8(rsgStates.STATE_PRE_READY);
elseif (state == uint8(rsgStates.STATE_ACQUIRE)) && acquiredTarget
    state = uint8(rsgStates.STATE_FIXATE);
    stateTimer = uint32(0);
    writeDiscreteData = true;
end

%%
%check for production trigger
distFromCenter = single(sqrt(sum(effectorPos.^2)));
productionTriggered = distFromCenter>cursorParameters.rsgFixationRadius;

if (state == uint8(rsgStates.STATE_PRE_READY)) || (state == uint8(rsgStates.STATE_POST_READY))
    if productionTriggered
        %illegal production time, fail
        lastSoundTime = clock;
        lastSoundState = uint8(SequenceStates.SOUND_STATE_FAIL);
        state = uint8(rsgStates.STATE_FIXATE);
    end
elseif (state == uint8(rsgStates.STATE_POST_SET))
    if productionTriggered
        %legal production time, measure reward
        producedTime = int32(stateTimer) - int32(cursorParameters.rsgCueDisplayTime);
        err = producedTime - int32(cursorParameters.rsgProductionTimes(trialIdx));
        
        percentErr = abs(single(err))/single(cursorParameters.rsgProductionTimes(trialIdx));
        totalErr = totalErr + percentErr;
        avgErr = totalErr/single(trialIdx);
        
        stateTimer = uint32(0);
        state = uint8(rsgStates.STATE_ACQUIRE);
        
        lastSoundTime = clock;
        lastSoundState = uint8(SequenceStates.SOUND_STATE_SUCCESS);
    end
end

%%
%timing
stateTimer = stateTimer + uint32(1);
if (state == uint8(rsgStates.STATE_PRE_READY)) 
    if stateTimer > cursorParameters.rsgPreReadyTimes(trialIdx);
        stateTimer = uint32(0);
        state = uint8(rsgStates.STATE_POST_READY);
    end
elseif (state == uint8(rsgStates.STATE_POST_READY)) 
    if stateTimer > (cursorParameters.rsgProductionTimes(trialIdx) + cursorParameters.rsgCueDisplayTime);
        stateTimer = uint32(0);
        state = uint8(rsgStates.STATE_POST_SET);
    end
end

%% PACK DATA FOR UDP OUTPUT (filelogger continuous)
taskOutput.continuous = packFileLoggerFormatAndData('continuous', ...
    TASK_NAME, VERSION_ID, ...
    'clock', clock, ...
    'blockNumber', stateParameters.blockNumber,...
    'pause', pauseTriggered, ...
    'xpcRequestClock', behaviorRequestClock, ...
    'peripheralTimestamp', peripheralTimestamp, ...
    'state', state, ...
    'inputType', inputType, ...
    'windowsMousePosition', behaviorPacket.windowsMousePosition, ...
    'windowsTimestamp', behaviorPacket.windowsTimestamp, ...
    'windowsPC1GazePoint', behaviorPacket.windowsPC1GazePoint, ...
    'windowsPC1GazePointValid', behaviorPacket.windowsPC1GazeValid, ...
    'windowsPC1HeadRot', behaviorPacket.windowsPC1HeadRot, ...
    'windowsPC1HeadRotValid', behaviorPacket.windowsPC1HeadRotValid, ...
    'windowsPC1Timestamp', behaviorPacket.windowsPC1Timestamp, ...
    'xpcScreenUpdateClock',vizPacket.xpcScreenUpdateClock,...
    'cursorPosition', single(effectorPos), ...
    'trialIdx', trialIdx, ...
    'stateTimer', stateTimer, ...
    'avgErr', avgErr,...
    'timeErr', err, ...   
    'producedTime', producedTime, ... 
    'targPos', targPos, ...  
    'targOverlap', targOverlap, ...  
    'cueDisplayTime', cursorParameters.rsgCueDisplayTime, ...
    'productionTime', cursorParameters.rsgProductionTimes(trialIdx), ...
    'preReadyTime', cursorParameters.rsgPreReadyTimes(trialIdx), ...
    'rsgFixationRadius', cursorParameters.rsgFixationRadius, ...
    'holdTime', cursorParameters.holdTime, ...
    'targetDiameter', cursorParameters.targetDiameter, ...
    'cursorDiameter', cursorParameters.cursorDiameter ...
);

%% SEND DISCRETE DATA TO FILELOGGER
workspaceAll = [cursorParameters.workspaceX; 
    cursorParameters.workspaceY;];

taskOutput.discrete = packFileLoggerFormatAndData('discrete', ...
    TASK_NAME, VERSION_ID, ...
    'clock', clock,...
    'blockNumber', stateParameters.blockNumber,...
    'taskType', cursorParameters.taskType, ...
    'inputType', inputType, ...
    'workspace', workspaceAll, ...    
    'outputType', outputType, ...
    'trialIdx', trialIdx, ...
    'avgErr', avgErr,...
    'timeErr', err, ...   
    'producedTime', producedTime, ...  
    'targPos', targPos, ...   
    'cueDisplayTime', cursorParameters.rsgCueDisplayTime, ...
    'productionTime', cursorParameters.rsgProductionTimes(trialIdx), ...
    'preReadyTime', cursorParameters.rsgPreReadyTimes(trialIdx), ...
    'rsgFixationRadius', cursorParameters.rsgFixationRadius, ...
    'holdTime', cursorParameters.holdTime, ...
    'targetDiameter', cursorParameters.targetDiameter, ...
    'cursorDiameter', cursorParameters.cursorDiameter ...
);

%% SEND DATA OUT TO VIZ
taskOutput.screen = packFileLoggerFormatAndData('screen', ...
    TASK_NAME, VERSION_ID, ...
    'clock', clock, ...
    'blockNumber', stateParameters.blockNumber,...
    'state', state, ...
    'cursorPosition', single(effectorPos), ...
    'trialIdx', trialIdx, ...
    'stateTimer', stateTimer, ...
    'avgErr', avgErr,...
    'timeErr', err, ...   
    'producedTime', producedTime, ... 
    'targPos', targPos, ...  
    'targOverlap', targOverlap, ...  
    'cueDisplayTime', cursorParameters.rsgCueDisplayTime, ...
    'productionTime', cursorParameters.rsgProductionTimes(trialIdx), ...
    'preReadyTime', cursorParameters.rsgPreReadyTimes(trialIdx), ...
    'rsgFixationRadius', cursorParameters.rsgFixationRadius, ...
    'holdTime', cursorParameters.holdTime, ...
    'targetDiameter', cursorParameters.targetDiameter, ...
    'cursorDiameter', cursorParameters.cursorDiameter ...
);

%% SEND DATA OUT TO SOUND
taskOutput.sound = packFileLoggerFormatAndData('screen', ...
    TASK_NAME, VERSION_ID, ...
    'clock', clock,...
    'vizState',state,...
    'err',err,...
    'lastSoundTime',lastSoundTime,...
    'lastSoundState',lastSoundState...
    ); 

%% SET SEND FLAGS FOR NETWORK OUTPUTS
if(clock < INIT_TIME)
    taskOutput.discrete.data.send = false;
    taskOutput.continuous.data.send = false;
    taskOutput.screen.data.send = false;
    taskOutput.sound.data.send = false;
    
    if(mod(clock, 10)==0)
        taskOutput.sendFormat = true;
    else
        taskOutput.sendFormat = false;
    end
else
    taskOutput.discrete.data.send = writeDiscreteData;
    taskOutput.continuous.data.send = writeContinuousData;
    taskOutput.screen.data.send = true;
    taskOutput.sound.data.send = true;
    taskOutput.sendFormat = false;
    taskOutput.inputType = inputType;
end
taskOutput.wiaCode = uint16(0);
taskOutput.speedCode = uint16(0);
taskOutput.paused = pauseTriggered;
taskOutput.clickTarget = uint16(0);
taskOutput.taskType = uint16(cursorParameters.taskType);

end

function vizPacket = parseVizPacket(packetData)
    vizPacket.xpcScreenUpdateClock = typecast(packetData(28+[1:4]), 'uint32');
end

function vizPacket = initVizPacket()
    vizPacket.xpcScreenUpdateClock = uint32(0);
end
